simulink model "H4Q_CPU"  (Simulink 8.1)
settings: Solver=FixedStepDiscrete  SolverMode=SingleTasking  StartTime=0.0  StopTime=inf  FixedStep=Ts  RelTol=1e-3
PostLoadFcn:
  | Init_Params;
InitFcn:
  | Init_Params;
undefined symbols (not defined in the file): I4Q, KLP4Q, P4Q, SatPIH4Q, TLP4Q, Tpas, Ts
libraries: rteventslib x6, simulink x5, rtlab x3, cpuconverter_lib x1, rtio_opalrt_common x1
settings Model: ARTEMISmethode_block_infos=$$__separator__$$  Creator=PYRobert  LastModifiedBy=Francis  BufferReuse=off
settings DataIOCC: SaveOutput=off  SignalLogging=off  SaveTime=off  SignalLoggingName=sigsOut
settings OptimizationCC: BlockReduction=off  OptimizeBlockIOStorage=off  BufferReuse=off  ExpressionFolding=off  LocalBlockOutputs=off  InitFltsAndDblsToZero=on
settings DebuggingCC: SaveWithParameterizedLinksMsg=none  SignalResolutionControl=TryResolveAllWithWarning  SolverPrmCheckMsg=none  MultiTaskDSMMsg=warning  MultiTaskCondExecSysMsg=none  StrictBusMsg=None
settings HardwareCC: TargetEndianess=LittleEndian  TargetHWDeviceType=MATLAB Host  ProdEqTarget=off
settings RTWCC: IncludeERTFirstTime=on
settings GRTTargetCC: TargetFcnLib=ansi_tfl_tmw.mat
settings ConfigurationSet: Description=SimMechanics 2G

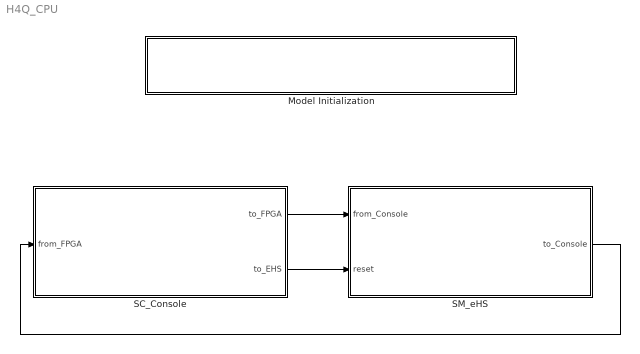
== system H4Q_CPU ==
  Model Initialization : Subsystem  mask(Model Functions){InitFcnX=Init_Params;, prel=off, posl=on, inif=on, strf=off}
      mask prompts: InitFcnX "Initialisation"; prel "Preload Function"; posl "PostLoad Function"; inif "InitFcn"; strf "StartFcn"
      mask init:
      | currentBlock = gcb;
      | root = bdroot(currentBlock);
      | 
      | if ~strcmp(get_param(root,'BlockDiagramType'),'library')
      |     if prel==1
      |         set_param(root, 'PreLoadFcn', InitFcnX);
      |     else
      |         set_param(root, 'PreLoadFcn', '');
      |     end
      |     if inif==1
      |         set_param(root, 'InitFcn', InitFcnX);
      |     else
      |         set_param(root, 'InitFcn', '');
      |     end
      |     if strf==1
      |         set_param(root, 'StartFcn', InitFcnX);
      |     else
      |         set_param(root, 'StartFcn', '');
      |     end
      |     if posl==1
      |         set_param(root, 'PostLoadFcn', InitFcnX);
      |     else
      |         set_param(root, 'PostLoadFcn', '');
      |     end
      | end
      | 
      | pos = get_param(currentBlock, 'Position');
      | width = pos(3) - pos(1); height = pos(4) - pos(2);
      | txt = [ upper(root) '\n' '- InitFcn. . . . . '  get_param(root, 'InitFcn') ];
      settings: CopyFcn=set_param(gcb,'LinkStatus','none')
      mask Display: text(5, height*0.5, txt, 'horizontalAlignment', 'left', 'verticalAlignment', 'middle') ;
  SC_Console : Subsystem
  SM_eHS : Subsystem
  wires:
  SC_Console/1(to_FPGA) -> SM_eHS/1(from_Console)
  SM_eHS/1(to_Console) -> SC_Console/1(from_FPGA)
  SC_Console/2(to_EHS) -> SM_eHS/2(reset)

== system H4Q_CPU/Model Initialization ==

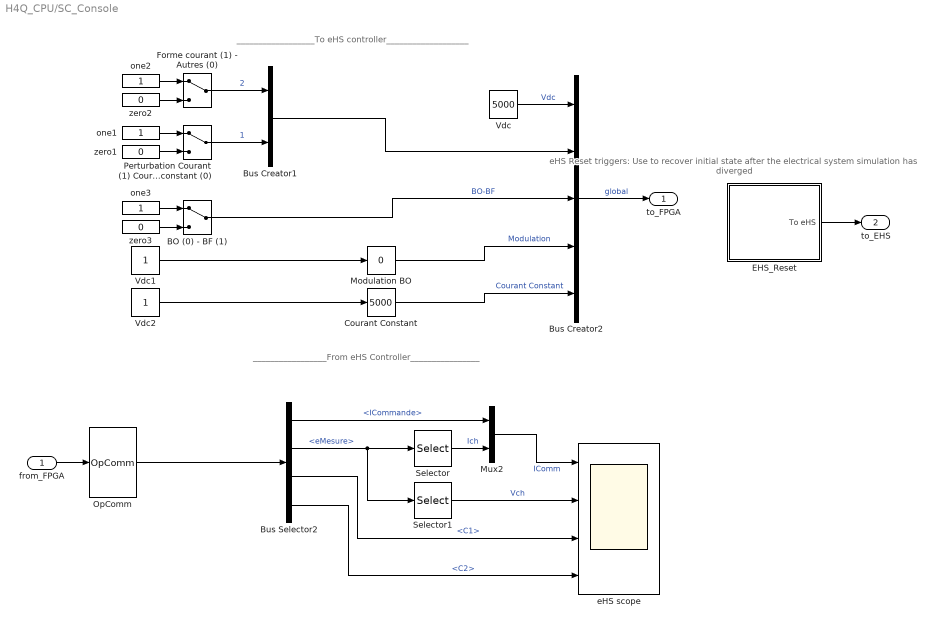
== system H4Q_CPU/SC_Console ==
  note: __________________To eHS controller___________________
  note: _________________From eHS Controller________________
  note: eHS Reset triggers:
      | Use to recover initial state after the
      | electrical system simulation has diverged
  from_FPGA : Inport
  BO (0) - BF (1) : ManualSwitch
  Bus Creator1 : BusCreator  Inputs=2
  Bus Creator2 : BusCreator  Inputs=5
  Bus Selector2 : BusSelector  OutputSignals=ICommande,eMesure,C1,C2
  Courant Constant : simulink/Math Operations/Slider Gain  low=-10000  gain=5000  high=10000
  EHS_Reset : Subsystem  mask(eHS settings){reset1=Reset Disabled}
      mask prompts: reset1 "Reset eHS1 :"
      mask TypeOptions reset1: Reset Disabled | Reset Enabled
  "Forme courant (1) - Autres (0) " : ManualSwitch
  Modulation BO : simulink/Math Operations/Slider Gain  low=-1  gain=0  high=1
  Mux2 : Mux  Inputs=2
  OpComm : rtlab/OpComm  nbport=1  groupe_acq=1  subsys_rate=0  st=0  Synchronization=off  Interpolation=off  Threshold=1.0  Missed_Data=off  Sim_Time=off  Samples=off  dynSigOut=off  from_console=0  warning_done=off  writeOpCommFile=off  Offset=off
  Perturbation Courant (1) Courant constant (0) : ManualSwitch
  Selector : Selector  IndexOptions=Index vector (dialog)  Indices=[1]  OutputSizes=1
  Selector1 : Selector  IndexOptions=Index vector (dialog)  Indices=[2]  OutputSizes=1
  Vdc : Constant  Value=5000
  Vdc1 : Constant
  Vdc2 : Constant
  eHS scope : Scope  NumInputPorts=4
      settings: TimeRange=0.9  YMin=0~-6000~-5~-5  YMax=7000~6000~5~5
  one1 : Constant
  one2 : Constant
  one3 : Constant
  zero1 : Constant  Value=0
  zero2 : Constant  Value=0
  zero3 : Constant  Value=0
  to_FPGA : Outport
  to_EHS : Outport  Port=2
  wires:
  Bus Creator2/1 -> to_FPGA/1  "global"
  Selector1/1 -> eHS scope/2  "Vch"
  EHS_Reset/1(To eHS) -> to_EHS/1
  Vdc/1 -> Bus Creator2/1  "Vdc"
  zero1/1 -> Perturbation Courant (1) Courant constant (0)/2
  one1/1 -> Perturbation Courant (1) Courant constant (0)/1
  zero2/1 -> "Forme courant (1) - Autres (0) "/2
  one2/1 -> "Forme courant (1) - Autres (0) "/1
  "Forme courant (1) - Autres (0) "/1 -> Bus Creator1/1  "2"
  Perturbation Courant (1) Courant constant (0)/1 -> Bus Creator1/2  "1"
  zero3/1 -> BO (0) - BF (1)/2
  one3/1 -> BO (0) - BF (1)/1
  Vdc1/1 -> Modulation BO/1
  Vdc2/1 -> Courant Constant/1
  from_FPGA/1 -> OpComm/1
  OpComm/1 -> Bus Selector2/1
  Bus Selector2/2 -> Selector/1, Selector1/1  "<eMesure>"
  Selector/1 -> Mux2/2  "Ich"
  Bus Selector2/1 -> Mux2/1  "<ICommande>"
  Mux2/1 -> eHS scope/1  "IComm"
  Bus Selector2/3 -> eHS scope/3  "<C1>"
  Bus Selector2/4 -> eHS scope/4  "<C2>"
  Bus Creator1/1 -> Bus Creator2/2
  BO (0) - BF (1)/1 -> Bus Creator2/3  "BO-BF"
  Modulation BO/1 -> Bus Creator2/4  "Modulation"
  Courant Constant/1 -> Bus Creator2/5  "Courant Constant"

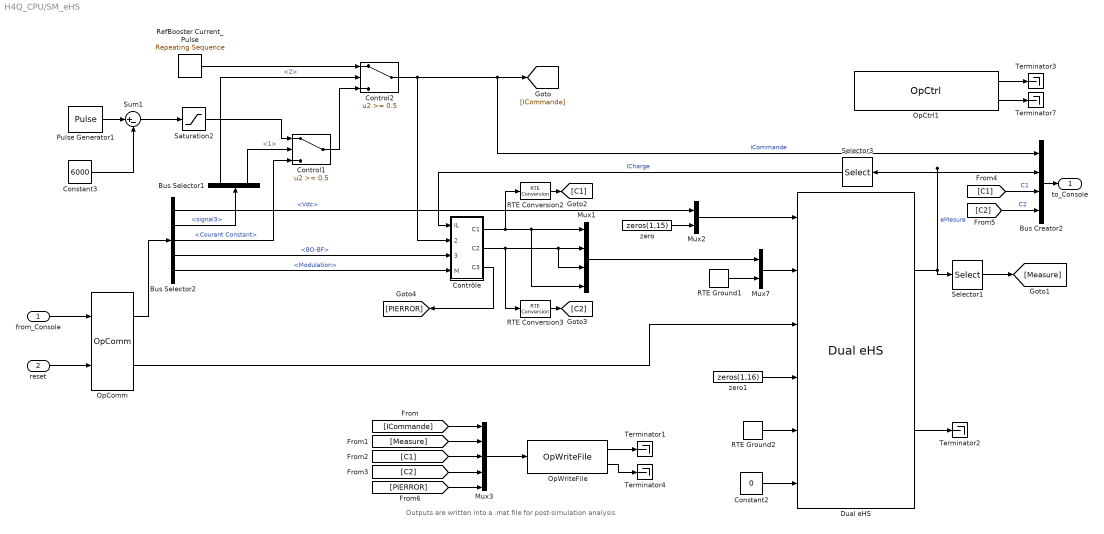
== system H4Q_CPU/SM_eHS ==
  note: Outputs are written into a .mat file
      | for post-simulation analysis
  from_Console : Inport
  reset : Inport  Port=2
  Bus Creator2 : BusCreator
  Bus Selector1 : BusSelector  OutputSignals=2,1
  Bus Selector2 : BusSelector  OutputSignals=Vdc,signal3,Courant Constant,BO-BF,Modulation
  Constant2 : Constant  Value=0
  Constant3 : Constant  Value=6000
  Control1 : Switch  Threshold=0.5
  Control2 : Switch  Threshold=0.5
  Contrôle : Subsystem  TreatAsAtomicUnit=on
      settings: MinAlgLoopOccurrences=on
  Dual eHS : cpuconverter_lib/Dual eHS  CtrlName='OpCtrl'  nb_eHS=1  nb_event=2  Ts=Ts  GenMat=off  circuit_mtx1=H4Q_FPGA  Pulse_ctrl1_popup=From RT-LAB block (all)  Pulse_ctrl1=zeros(1,24)  Polarity1_popup=Active-high (all)  Polarity1=zeros(1,24)  Ts_eHS_1_explicit=off  Ts_eHS_1=1.2e-007  Input_config1_popup=From RT-LAB block (all)  input_config_1=zeros(1,16)  SimeHS1=off  blkid1=1e-007  ShowAdv1=on  gs1=0.01  v_init1=zeros(1,24)  i_init1=zeros(1,24)  circuit_mtx2=RC_std2  Pulse_ctrl2_popup=Independent setting for each element  Pulse_ctrl2=0  Polarity2_popup=Active-high (all)  Polarity2=zeros(1,24)  Ts_eHS_2_explicit=off  Ts_eHS_2=1.2e-007  Input_config2_popup=Independent setting for each element  input_config_2=0  blkid2=0  ShowAdv2=on  gs2=1  v_init2=zeros(1,24)  i_init2=zeros(1,24)  PortNbs=[1 2 3 1 2 5 6 7 8 9 10 1 2]  UseSWG=off  SWGPortNbs=[4 5]
      settings: AttributesFormatString=%<CtrlName>
  Mux1 : Mux
  Mux2 : Mux  Inputs=[1 15]
  Mux3 : Mux  Inputs=[1 2 1 1 2]
  Mux7 : Mux  Inputs=[4 -1]
  OpComm : rtlab/OpComm  nbport=2  groupe_acq=1  subsys_rate=0  st=0  Synchronization=on  Interpolation=on  Threshold=1.0  Missed_Data=off  Sim_Time=off  Samples=off  dynSigOut=off  from_console=1  warning_done=off  writeOpCommFile=off  Offset=off
  OpCtrl1 : rtio_opalrt_common/OpCtrl  CtrlName='OpCtrl'  boardid=0  BitstreamFilename=MMPK7_1-EX-0001-2_2_2_41-2_eHS_std_noIO-03-1D.bin  numconfig=-1  mode=Master  externalClock=off  decimRtsi=0  calibIO=off  SampleTime=0  loadinport=-1  BoardType=OP4500  SecondaryPresent=off  sync_type=Audio
  OpWriteFile : rtlab/DataLogging/OpWriteFile  Static_File=on  Nb_Samples=0.001/25e-6  Buffer_size=0.1/25e-6 * 8 * 8  Filename=myfile2.mat  varname=opvar2  Sim_Mode=off  Acq_Group=26  file_size=3/25e-6 * 8 * 3  write_offline=off
  Pulse Generator1 : DiscretePulseGenerator  Amplitude=12000  Period=floor(.4 /Tpas)  PulseWidth=floor(.4 * .5 / Tpas)  PhaseDelay=floor(.001 / Tpas)  SampleTime=Tpas
  RTE Conversion2 : rteventslib/Signal Attributes/RTE Conversion  inputdatatype=RTE Boolean  outputdatatype=Double  compensation=Enabled  nbMaxEvents=10  sampleTime=Ts
  RTE Conversion3 : rteventslib/Signal Attributes/RTE Conversion  inputdatatype=RTE Boolean  outputdatatype=Double  compensation=Enabled  nbMaxEvents=10  sampleTime=Ts
  RTE Ground1 : rteventslib/Sources/RTE Ground  SampleTime=Ts
  RTE Ground2 : rteventslib/Sources/RTE Ground  SampleTime=Ts
  RefBooster Current_Pulse : simulink/Sources/Repeating Sequence  rep_seq_t="[0 108.51e-3 127.6e-3 132e-3 200e-3 250e-3 283.33e-3 310e-3 366.66e-3  490e-3 533e-3 683.33e-3 900e-3]"  rep_seq_y=[333 333 1000 1031 1500 2000 2500 3000 4000 6000 6000 333 333]
  Saturation2 : Saturate  UpperLimit=5000  LowerLimit=2000
  Selector1 : Selector  IndexOptions=Index vector (dialog)  Indices=[1 2]  OutputSizes=1
  Selector3 : Selector  IndexOptions=Index vector (dialog)  Indices=[1]  OutputSizes=1
  Sum1 : Sum  Inputs=|+-
  Terminator{1..4,7} (5 alike) : Terminator
  zero : Constant  Value=zeros(1,15)
  zero1 : Constant  Value=zeros(1,16)
  to_Console : Outport
  wires:
  from_Console/1 -> OpComm/1
  Mux2/1 -> Dual eHS/1
  Dual eHS/1 -> Selector1/1, Selector3/1, Bus Creator2/2  "eMesure"
  Mux7/1 -> Dual eHS/2
  RTE Ground1/1 -> Mux7/2
  reset/1 -> OpComm/2
  Bus Selector2/1 -> Mux2/1  "<Vdc>"
  zero/1 -> Mux2/2
  Mux1/1 -> Mux7/1
  OpCtrl1/1 -> Terminator3/1
  OpCtrl1/2 -> Terminator7/1
  zero1/1 -> Dual eHS/4
  RTE Ground2/1 -> Dual eHS/5
  Constant2/1 -> Dual eHS/6
  OpComm/2 -> Dual eHS/3
  Dual eHS/2 -> Terminator2/1
  Contrôle/2(C2) -> Mux1/2, Mux1/3, RTE Conversion3/1
  Contrôle/1(C1) -> Mux1/4, Mux1/1, RTE Conversion2/1
  Selector3/1 -> Contrôle/1(IL)  "ICharge"
  Saturation2/1 -> Control1/1
  Constant3/1 -> Sum1/2
  RefBooster Current_Pulse/1 -> Control2/1
  Control1/1 -> Control2/3
  Pulse Generator1/1 -> Sum1/1
  Sum1/1 -> Saturation2/1
  Control2/1 -> Contrôle/2(Iref), Bus Creator2/1, [ICommande]  "ICommande"
  Bus Selector2/2 -> Bus Selector1/1  "<signal3>"
  Bus Selector2/4 -> Contrôle/3(BO/BF)  "<BO-BF>"
  Bus Selector2/5 -> Contrôle/4(M)  "<Modulation>"
  Bus Selector1/2 -> Control1/2  "<1>"
  Bus Selector1/1 -> Control2/2  "<2>"
  Bus Selector2/3 -> Control1/3  "<Courant Constant>"
  Bus Creator2/1 -> to_Console/1
  OpComm/1 -> Bus Selector2/1
  [ICommande] -> Mux3/1
  OpWriteFile/1 -> Terminator1/1
  OpWriteFile/2 -> Terminator4/1
  Selector1/1 -> [Measure]
  [Measure] -> Mux3/2
  [C1] -> Mux3/3
  [C2] -> Mux3/4
  [C1] -> Bus Creator2/3  "C1"
  [C2] -> Bus Creator2/4  "C2"
  RTE Conversion2/1 -> [C1]
  RTE Conversion3/1 -> [C2]
  Contrôle/3(C3) -> [PIERROR]
  Mux3/1 -> OpWriteFile/1
  [PIERROR] -> Mux3/5

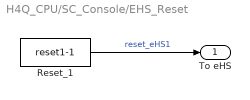
== system H4Q_CPU/SC_Console/EHS_Reset ==
  Reset_1 : Constant  Value=reset1-1
  To eHS : Outport
  wires:
  Reset_1/1 -> To eHS/1  "reset_eHS1"

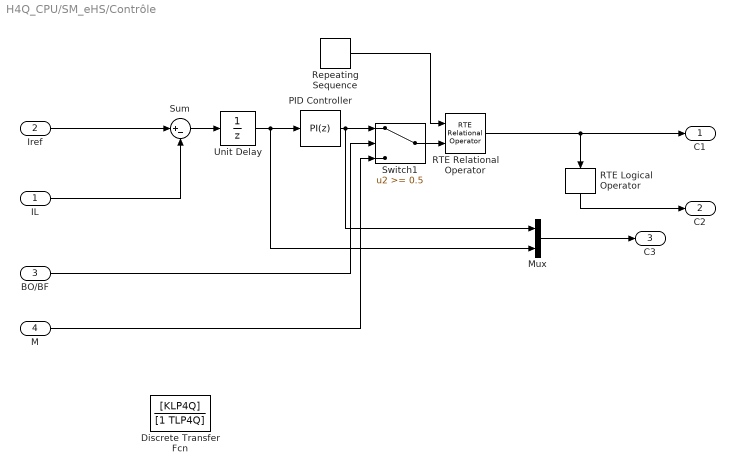
== system H4Q_CPU/SM_eHS/Contrôle ==
  IL : Inport
  Iref : Inport  Port=2
  BO/BF : Inport  Port=3
  M : Inport  Port=4
  Discrete Transfer Fcn : DiscreteTransferFcn  Numerator=[KLP4Q]  Denominator=[1 TLP4Q]  SampleTime=Tpas
  Mux : Mux  Inputs=2
  PID Controller : simulink/Continuous/PID Controller  Controller=PI  TimeDomain=Discrete-time  SampleTime=Tpas  IntegratorMethod=Forward Euler  FilterMethod=Forward Euler  Form=Parallel  P=P4Q  I=I4Q  D=0  N=100  InitialConditionSource=internal  InitialConditionForIntegrator=0  InitialConditionForFilter=0  ExternalReset=none  LimitOutput=on  UpperSaturationLimit=SatPIH4Q  LowerSaturationLimit=-SatPIH4Q  LinearizeAsGain=on  AntiWindupMode=clamping  Kb=1  TrackingMode=off  Kt=1  PParamMin=[]  PParamMax=[]  IParamMin=[]  IParamMax=[]  DParamMin=[]  DParamMax=[]  NParamMin=[]  NParamMax=[]  KbParamMin=[]  KbParamMax=[]  KtParamMin=[]  KtParamMax=[]  POutMin=[]  POutMax=[]  IOutMin=[]  IOutMax=[]  DOutMin=[]  DOutMax=[]  NOutMin=[]  NOutMax=[]  KbOutMin=[]  KbOutMax=[]  KtOutMin=[]  KtOutMax=[]  IntegratorOutMin=[]  IntegratorOutMax=[]  FilterOutMin=[]  FilterOutMax=[]  SumOutMin=[]  SumOutMax=[]  SumI1OutMin=[]  SumI1OutMax=[]  SumI2OutMin=[]  SumI2OutMax=[]  SumI3OutMin=[]  SumI3OutMax=[]  SumDOutMin=[]  SumDOutMax=[]  SaturationOutMin=[]  SaturationOutMax=[]  IntegratorContinuousStateAttributes=''  IntegratorStateMustResolveToSignalObject=off  IntegratorRTWStateStorageClass=Auto  FilterContinuousStateAttributes=''  FilterStateMustResolveToSignalObject=off  FilterRTWStateStorageClass=Auto
  RTE Logical Operator : rteventslib/Math Operations/RTE Logical Operator  LogicalOperator=NOT  NbrInput=1  NbrMaxEvents=10
  RTE Relational Operator : rteventslib/Math Operations/RTE Relational Operator  RelationalOperator=<  NumberMaxEvents=1  SampleTime=Tpas
  Repeating Sequence : simulink/Sources/Repeating Sequence  rep_seq_t=[0 1e-3/2 1e-3]  rep_seq_y=[1 -1 1]
  Sum : Sum  Inputs=|+-
  Switch1 : Switch  Threshold=0.5
  Unit Delay : UnitDelay  SampleTime=-1
  C1 : Outport
  C2 : Outport  Port=2
  C3 : Outport  Port=3
  wires:
  Repeating Sequence/1 -> RTE Relational Operator/1
  RTE Relational Operator/1 -> RTE Logical Operator/1, C1/1
  RTE Logical Operator/1 -> C2/1
  IL/1 -> Sum/2
  Iref/1 -> Sum/1
  Sum/1 -> Unit Delay/1
  Switch1/1 -> RTE Relational Operator/2
  PID Controller/1 -> Switch1/1, Mux/1
  BO/BF/1 -> Switch1/2
  M/1 -> Switch1/3
  Mux/1 -> C3/1
  Unit Delay/1 -> PID Controller/1, Mux/2
